simulink model "LQR_longitudinal"  (R2016b)
settings: Solver=VariableStepAuto  StartTime=0.0  StopTime=20  RelTol=1e-3
undefined symbols (not defined in the file or in its folder): A_long, B_long, C_long, K_long
libraries: dspsrcs4 x1
settings Model: Creator=yashm  LastModifiedBy=yashm

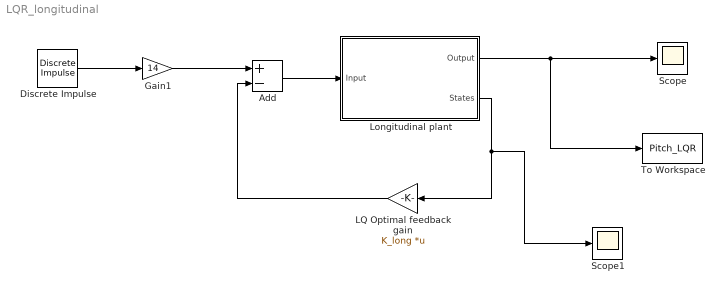
== system LQR_longitudinal ==
  Add : Sum  Inputs=+-
  Discrete Impulse : dspsrcs4/Discrete  Impulse  Delay=0  SampleTime=1  FrameSample=1  OutputFrames=off  dataType=double  isSigned=on  wordLen=16  udDataType=sfix(16)  fracBitsMode=Best precision  numFracBits=15  OutDataTypeStr=double  LastOutDataTypeStr=double
  Gain1 : Gain  Gain=14
  LQ Optimal feedback gain : Gain  Gain=K_long  Multiplication=Matrix(K*u)
  Longitudinal plant : Subsystem
  Scope : Scope
  Scope1 : Scope
  To Workspace : ToWorkspace  VariableName=Pitch_LQR  SampleTime=0.4
      settings: Save2DSignal=2-D array (concatenate along first dimension)
  wires:
  Longitudinal plant/1(Output) -> Scope/1, To Workspace/1
  Add/1 -> Longitudinal plant/1(Input)
  Longitudinal plant/2(States) -> Scope1/1, LQ Optimal feedback gain/1
  LQ Optimal feedback gain/1 -> Add/2
  Gain1/1 -> Add/1
  Discrete Impulse/1 -> Gain1/1

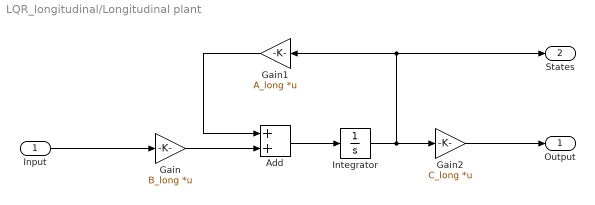
== system LQR_longitudinal/Longitudinal plant ==
  Input : Inport
  Add : Sum
  Gain : Gain  Gain=B_long  Multiplication=Matrix(K*u)
  Gain1 : Gain  Gain=A_long  Multiplication=Matrix(K*u)
  Gain2 : Gain  Gain=C_long  Multiplication=Matrix(K*u)
  Integrator : Integrator  InitialCondition=[0 0 10]
  Output : Outport
  States : Outport  Port=2
  wires:
  Gain2/1 -> Output/1
  Input/1 -> Gain/1
  Gain/1 -> Add/2
  Integrator/1 -> Gain1/1, States/1, Gain2/1
  Add/1 -> Integrator/1
  Gain1/1 -> Add/1
